simulink model "RcvyLStateCtrl"  (R2018b)
settings: Solver=FixedStepDiscrete  StartTime=0.0  StopTime=10.0  FixedStep=0.01  RelTol=1e-3
libraries: StateCtrlLib x1
settings Model: Creator=sn2xws  LastModifiedBy=sn2xws
settings DataIOCC: SaveFormat=StructureWithTime
settings OptimizationCC: DefaultParameterBehavior=Inlined  EnhancedBackFolding=on  PassReuseOutputArgsAs=Individual arguments  ZeroExternalMemoryAtStartup=off  ZeroInternalMemoryAtStartup=off  OptimizeBlockOrder=speed  DifferentSizesBufferReuse=on  OptimizationCustomize=off
settings DebuggingCC: ParameterTunabilityLossMsg=error
settings ModelReferenceCC: ModelReferenceNumInstancesAllowed=Single
settings SFSimCC: MATLABDynamicMemAlloc=off
settings RTWCC: SystemTargetFile=autosar.tlc  GenCodeOnly=on  TemplateMakefile=ert_default_tmf  Description=AUTOSAR  GenerateReport=on  IncludeHyperlinkInReport=on  LaunchReport=on  GenerateTraceInfo=on  GenerateTraceReport=on  GenerateTraceReportSl=on  GenerateTraceReportSf=on  GenerateTraceReportEml=on
settings CodeAppCC: ForceParamTrailComments=on  IgnoreCustomStorageClasses=off  OperatorAnnotations=on  SimulinkDataObjDesc=on  SFDataObjDesc=on  InsertBlockDesc=on
settings STFCustomTargetCC: TargetLangStandard=C99 (ISO)  MultiwordLength=256  ParMdlRefBuildCompliant=on  CompOptLevelCompliant=on  IncludeMdlTerminateFcn=off  CombineOutputUpdateFcns=on  SuppressErrorStatus=on  ERTCustomFileBanners=on  SupportNonFinite=off  SupportComplex=off  SupportContinuousTime=off  SupportNonInlinedSFcns=off  RemoveResetFunc=on  MATLABClassNameForMDSCustomization=Simulink.SoftwareTarget.ERTCustomization  AutosarCompliant=on  UseToolchainInfoCompliant=on  LookupTableObjectStructAxisOrder=2,1,3,4,...  LUTObjectStructOrderEvenSpacing=Size,Table,Breakpoints  SystemTargetFile=autosar.tlc
settings ERTTargetCC: TargetLangStandard=C99 (ISO)  ConcurrentExecutionCompliant=off  IncludeMdlTerminateFcn=off  SuppressErrorStatus=on  SupportNonFinite=off  SupportComplex=off  ModelStepFunctionPrototypeControlCompliant=off  CPPClassGenCompliant=off  AutosarCompliant=on  LookupTableObjectStructAxisOrder=2,1,3,4,...  LUTObjectStructOrderEvenSpacing=Size,Table,Breakpoints  InlinedParameterPlacement=NonHierarchical  ERTCustomFileTemplate=example_file_process.tlc

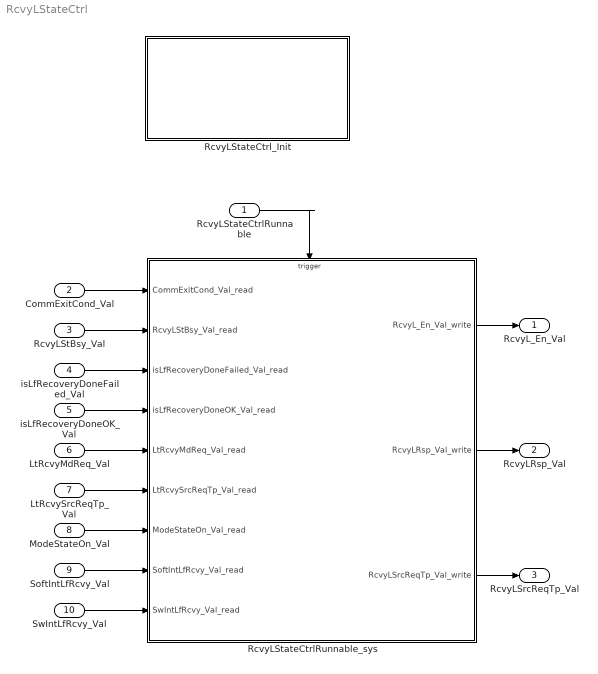
== system RcvyLStateCtrl ==
  RcvyLStateCtrlRunnable : Inport  SampleTime=0.01  OutputFunctionCall=on
  CommExitCond_Val : Inport  Port=2  OutDataTypeStr=boolean  PortDimensions=1
  RcvyLStBsy_Val : Inport  Port=3  OutDataTypeStr=boolean  PortDimensions=1
  isLfRecoveryDoneFailed_Val : Inport  Port=4  OutDataTypeStr=boolean  PortDimensions=1
  isLfRecoveryDoneOK_Val : Inport  Port=5  OutDataTypeStr=boolean  PortDimensions=1
  LtRcvyMdReq_Val : Inport  Port=6  OutDataTypeStr=boolean  PortDimensions=1
  LtRcvySrcReqTp_Val : Inport  Port=7  OutDataTypeStr=Enum: SrcReqTp1  PortDimensions=1
  ModeStateOn_Val : Inport  Port=8  OutDataTypeStr=boolean  PortDimensions=1
  SoftIntLfRcvy_Val : Inport  Port=9  OutDataTypeStr=IntEnable  PortDimensions=1
  SwIntLfRcvy_Val : Inport  Port=10  OutDataTypeStr=IntEnable  PortDimensions=1
  RcvyLStateCtrlRunnable_sys : Subsystem
  RcvyLStateCtrl_Init : Subsystem
  RcvyL_En_Val : Outport  OutDataTypeStr=boolean  PortDimensions=1
  RcvyLRsp_Val : Outport  Port=2  OutDataTypeStr=Enum: MdRspLocal1  PortDimensions=1
  RcvyLSrcReqTp_Val : Outport  Port=3  OutDataTypeStr=Enum: SrcReqTp1  PortDimensions=1
  wires:
  CommExitCond_Val/1 -> RcvyLStateCtrlRunnable_sys/1(CommExitCond_Val_read)
  RcvyLStBsy_Val/1 -> RcvyLStateCtrlRunnable_sys/2(RcvyLStBsy_Val_read)
  isLfRecoveryDoneFailed_Val/1 -> RcvyLStateCtrlRunnable_sys/3(isLfRecoveryDoneFailed_Val_read)
  isLfRecoveryDoneOK_Val/1 -> RcvyLStateCtrlRunnable_sys/4(isLfRecoveryDoneOK_Val_read)
  LtRcvyMdReq_Val/1 -> RcvyLStateCtrlRunnable_sys/5(LtRcvyMdReq_Val_read)
  LtRcvySrcReqTp_Val/1 -> RcvyLStateCtrlRunnable_sys/6(LtRcvySrcReqTp_Val_read)
  ModeStateOn_Val/1 -> RcvyLStateCtrlRunnable_sys/7(ModeStateOn_Val_read)
  SoftIntLfRcvy_Val/1 -> RcvyLStateCtrlRunnable_sys/8(SoftIntLfRcvy_Val_read)
  SwIntLfRcvy_Val/1 -> RcvyLStateCtrlRunnable_sys/9(SwIntLfRcvy_Val_read)
  RcvyLStateCtrlRunnable_sys/1(RcvyL_En_Val_write) -> RcvyL_En_Val/1
  RcvyLStateCtrlRunnable_sys/2(RcvyLRsp_Val_write) -> RcvyLRsp_Val/1
  RcvyLStateCtrlRunnable_sys/3(RcvyLSrcReqTp_Val_write) -> RcvyLSrcReqTp_Val/1
  RcvyLStateCtrlRunnable/1 -> RcvyLStateCtrlRunnable_sys/Trigger

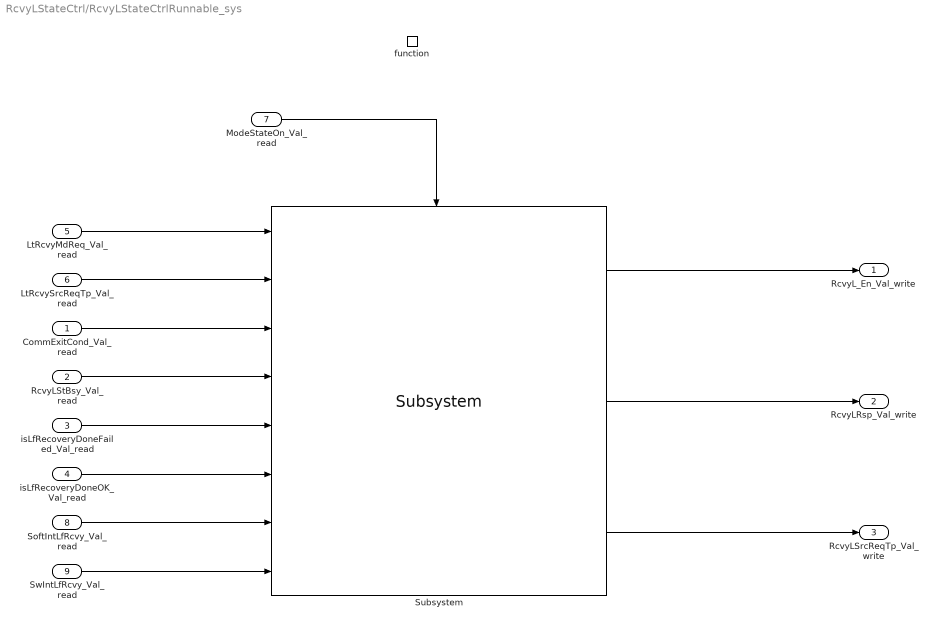
== system RcvyLStateCtrl/RcvyLStateCtrlRunnable_sys ==
  CommExitCond_Val_read : Inport
  RcvyLStBsy_Val_read : Inport  Port=2
  isLfRecoveryDoneFailed_Val_read : Inport  Port=3
  isLfRecoveryDoneOK_Val_read : Inport  Port=4
  LtRcvyMdReq_Val_read : Inport  Port=5
  LtRcvySrcReqTp_Val_read : Inport  Port=6
  ModeStateOn_Val_read : Inport  Port=7
  SoftIntLfRcvy_Val_read : Inport  Port=8  OutDataTypeStr=IntEnable
  SwIntLfRcvy_Val_read : Inport  Port=9  OutDataTypeStr=IntEnable
  function : TriggerPort  TriggerType=function-call  VariantControl=(inherit)  SampleTimeType=periodic  SampleTime=-1
  Subsystem : StateCtrlLib/Subsystem  SystemSampleTime=-1
  RcvyL_En_Val_write : Outport
      settings: EnsureOutportIsVirtual=on
  RcvyLRsp_Val_write : Outport  Port=2
      settings: EnsureOutportIsVirtual=on
  RcvyLSrcReqTp_Val_write : Outport  Port=3
      settings: EnsureOutportIsVirtual=on
  wires:
  Subsystem/3 -> RcvyLSrcReqTp_Val_write/1
  Subsystem/2 -> RcvyLRsp_Val_write/1
  Subsystem/1 -> RcvyL_En_Val_write/1
  ModeStateOn_Val_read/1 -> Subsystem/Enable
  LtRcvyMdReq_Val_read/1 -> Subsystem/1
  LtRcvySrcReqTp_Val_read/1 -> Subsystem/2
  CommExitCond_Val_read/1 -> Subsystem/3
  RcvyLStBsy_Val_read/1 -> Subsystem/4
  isLfRecoveryDoneFailed_Val_read/1 -> Subsystem/5
  isLfRecoveryDoneOK_Val_read/1 -> Subsystem/6
  SoftIntLfRcvy_Val_read/1 -> Subsystem/7
  SwIntLfRcvy_Val_read/1 -> Subsystem/8

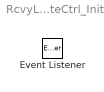
== system RcvyLStateCtrl/RcvyLStateCtrl_Init ==
  Event Listener : EventListener  EventName=reset
